simulink model "main"  (R2019b)
settings: Solver=VariableStepAuto  StartTime=0.0  StopTime=3  RelTol=1e-6  EnableMultiTasking=on
values from neighbouring files (symbols this model uses):
  gamma = 1.4    [main.m]
  M = kron(eye(N),C)    [MpcVectorize.m]    (also in MpcVectorizeLinearized.m; main.m = [0 1 0; 0 0 0])
  m = 1    [main.m]
  N = 20    [main.m]
  n = 3    [main.m]
  PI_Linear = 0.99    [main.m]
  q1 = [1e8 0; 0 0]    [main.m]
  q2 = 1e-8    (= 1e-08)    [main.m]
  Ts = 0.01    [main.m]
  x0 = [0.177; 2e4; 0]    [main.m]
  x0_plant = [0.177; 2e4]    [main.m]
undefined symbols (not defined in the file or in its folder): ENGINE, PI_Input
libraries: simulink x1, powerlib_meascontrol x1
settings Model: Creator=Robin  LastModifiedBy=geoja551
settings DataIOCC: ReturnWorkspaceOutputs=off
settings OptimizationCC: LifeSpan=inf
settings DebuggingCC: SFUnexpectedBacktrackingDiag=warning  SFNoUnconditionalDefaultTransitionDiag=warning  UnderSpecifiedDimensionMsg=warning  ArithmeticOperatorsInVariantConditions=warning
settings SFSimCC: SimUseLocalCustomCode=off  CustomCodeUndefinedFunction=UseInterfaceOnly
settings RTWCC: RTWUseLocalCustomCode=off
settings CodeAppCC: StateflowObjectComments=on
settings GRTTargetCC: TargetLangStandard=C89/C90 (ANSI)  GeneratePreprocessorConditionals=Disable all
settings ConfigComp: CovMetricSettings=dw  CovHtmlReporting=on  CovSaveCumulativeToWorkspaceVar=on  CovSaveSingleToWorkspaceVar=on  CovExternalEMLEnable=off

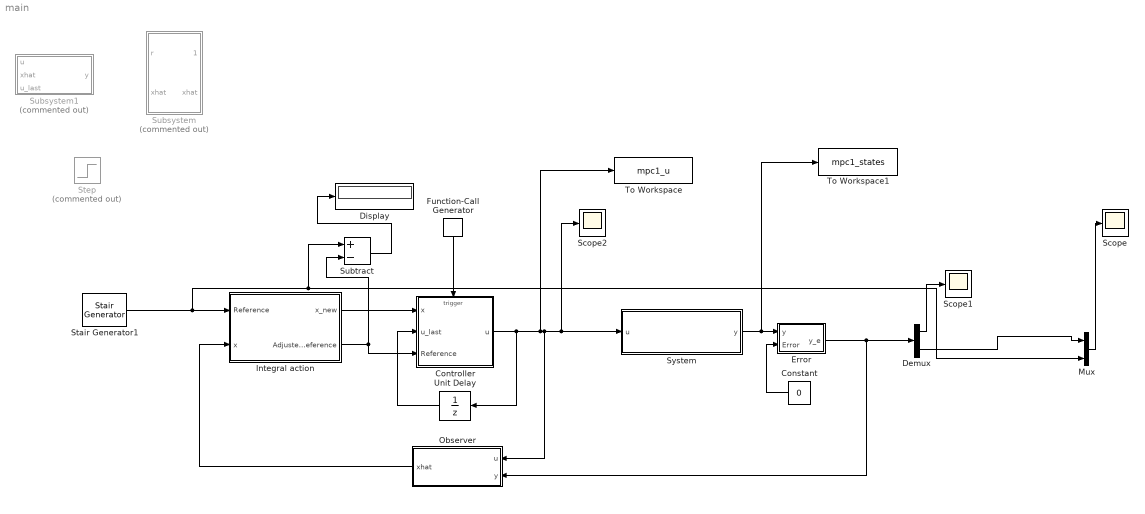
== system main ==
  Constant : Constant  Value=0
  Controller : Subsystem
  Demux : Demux  Outputs=2
  Display : Display
  Error : Subsystem
  Function-Call Generator : simulink/Ports & Subsystems/Function-Call Generator  sample_time=Ts  numberOfIterations=1
  Integral action : Subsystem
  Mux : Mux  Inputs=2
  Observer : Subsystem
  Scope : Scope
  Scope1 : Scope
  Scope2 : Scope
  Stair Generator1 : powerlib_meascontrol/Pulse & Signal Generators/Stair Generator  t=[0,1]  e=[ 2e4,8e4]  Ts=0
      settings: SourceProductName=Simscape Electrical
  Step : Step  Commented=on  Time=4  Before=2e4  After=6e4  SampleTime=0
  Subsystem : Subsystem  Commented=on
  Subsystem1 : Subsystem  Commented=on
  Subtract : Sum  Inputs=+-
  System : Subsystem
  To Workspace : ToWorkspace  VariableName=mpc1_u  SaveFormat=Structure With Time  SampleTime=-1
  To Workspace1 : ToWorkspace  VariableName=mpc1_states  SaveFormat=Structure With Time  SampleTime=-1
  Unit Delay : UnitDelay  InitialCondition=x0(1)  SampleTime=Ts  HasFrameUpgradeWarning=on
  wires:
  Function-Call Generator/1 -> Controller/Trigger
  Unit Delay/1 -> Controller/2(u_last)
  Controller/1(u) -> To Workspace/1, Scope2/1, System/1(u), Observer/1(u), Unit Delay/1
  System/1(y) -> To Workspace1/1, Error/1(y)
  Error/1(y_e) -> Demux/1, Observer/2(y)
  Constant/1 -> Error/2(Error)
  Integral action/2(Adjusted Reference) -> Subtract/2, Controller/3(Reference)
  Observer/1(xhat) -> Integral action/2(x)
  Integral action/1(x_new) -> Controller/1(x)
  Demux/2 -> Mux/1
  Demux/1 -> Scope1/1
  Mux/1 -> Scope/1
  Stair Generator1/1 -> Subtract/1, Mux/2, Integral action/1(Reference)
  Subtract/1 -> Display/1

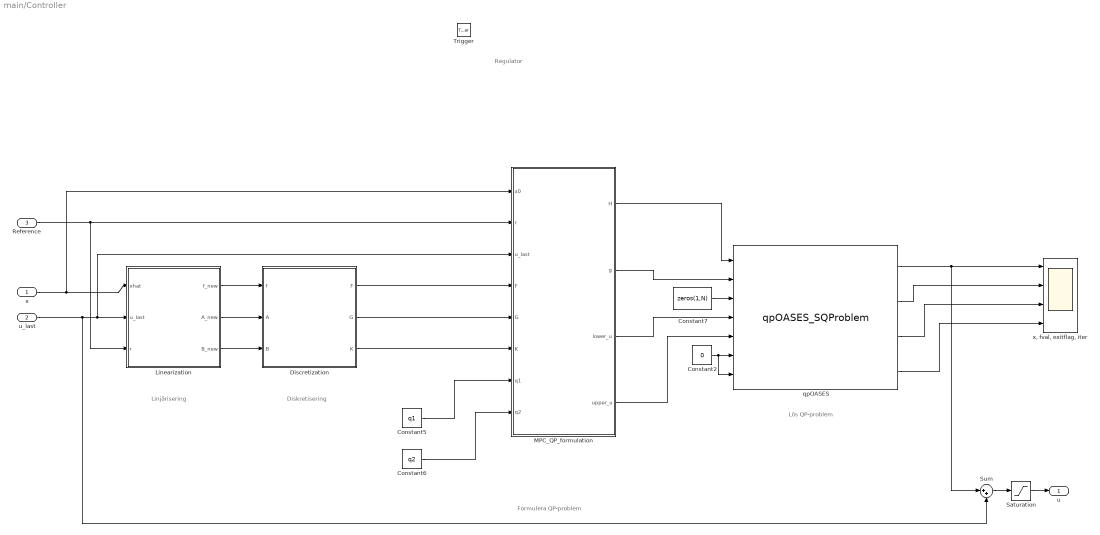
== system main/Controller ==
  note: Diskretisering
  note: Regulator
  note: Formulera QP-problem
  note: Lös QP-problem
  note: Linjärisering
  x : Inport
  u_last : Inport  Port=2  PortDimensions=1
  Reference : Inport  Port=3
  Trigger : TriggerPort  TriggerType=function-call  VariantControl=Variant  PortDimensions=1
  Constant2 : Constant  Value=0
  Constant5 : Constant  Value=q1
  Constant6 : Constant  Value=q2
  Constant7 : Constant  Value=zeros(1,N)
  Discretization : MATLAB Function  TreatAsAtomicUnit=on
  Linearization : MATLAB Function  TreatAsAtomicUnit=on
  MPC_QP_formulation : MATLAB Function  TreatAsAtomicUnit=on
  Saturation : Saturate  UpperLimit=1  LowerLimit=0
  Sum : Sum  Inputs=|++
  qpOASES : S-Function  FunctionName=qpOASES_SQProblem  SFunctionDeploymentMode=off  EnableBusSupport=off
  "x, fval, exitflag, iter" : Scope  NumInputPorts=4
  u : Outport
  wires:
  Linearization/2(A_new) -> Discretization/2(A)
  Linearization/3(B_new) -> Discretization/3(B)
  Discretization/1(F) -> MPC_QP_formulation/4(F)
  Discretization/2(G) -> MPC_QP_formulation/5(G)
  Constant6/1 -> MPC_QP_formulation/8(q2)
  Constant5/1 -> MPC_QP_formulation/7(q1)
  qpOASES/1 -> Sum/1, "x, fval, exitflag, iter"/1
  qpOASES/2 -> "x, fval, exitflag, iter"/2
  qpOASES/3 -> "x, fval, exitflag, iter"/3
  qpOASES/4 -> "x, fval, exitflag, iter"/4
  MPC_QP_formulation/2(g) -> qpOASES/2
  Constant7/1 -> qpOASES/3
  MPC_QP_formulation/3(lower_u) -> qpOASES/4
  MPC_QP_formulation/4(upper_u) -> qpOASES/5
  MPC_QP_formulation/1(H) -> qpOASES/1
  Constant2/1 -> qpOASES/7, qpOASES/6
  x/1 -> MPC_QP_formulation/1(x0), Linearization/1(xhat)
  u_last/1 -> Sum/2, Linearization/2(u_last), MPC_QP_formulation/3(u_last)
  Discretization/3(K) -> MPC_QP_formulation/6(K)
  Reference/1 -> Linearization/3(r), MPC_QP_formulation/2(r)
  Linearization/1(f_new) -> Discretization/1(f)
  Saturation/1 -> u/1
  Sum/1 -> Saturation/1

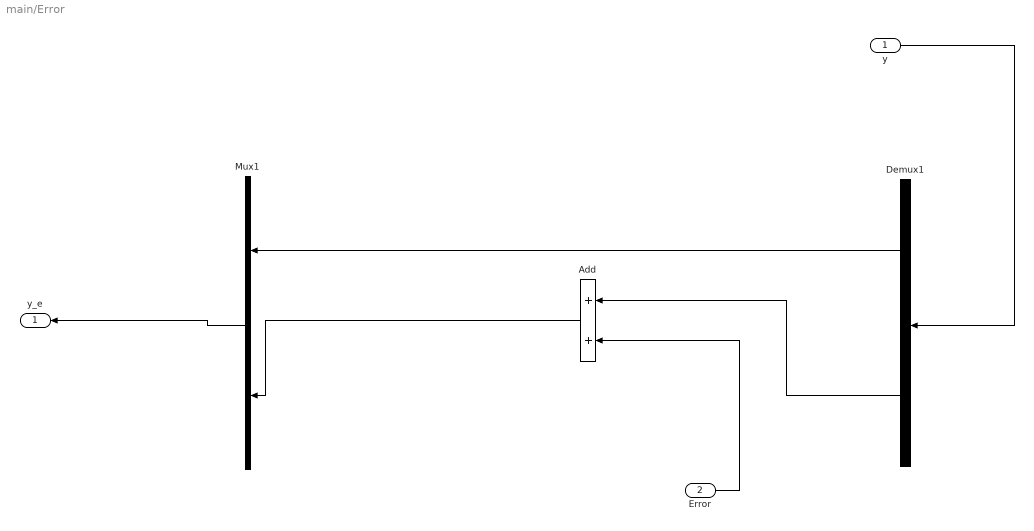
== system main/Error ==
  y : Inport
  Error : Inport  Port=2
  Add : Sum
  Demux1 : Demux  Outputs=2
  Mux1 : Mux  Inputs=2
  y_e : Outport
  wires:
  y/1 -> Demux1/1
  Mux1/1 -> y_e/1
  Demux1/2 -> Add/1
  Add/1 -> Mux1/2
  Demux1/1 -> Mux1/1
  Error/1 -> Add/2

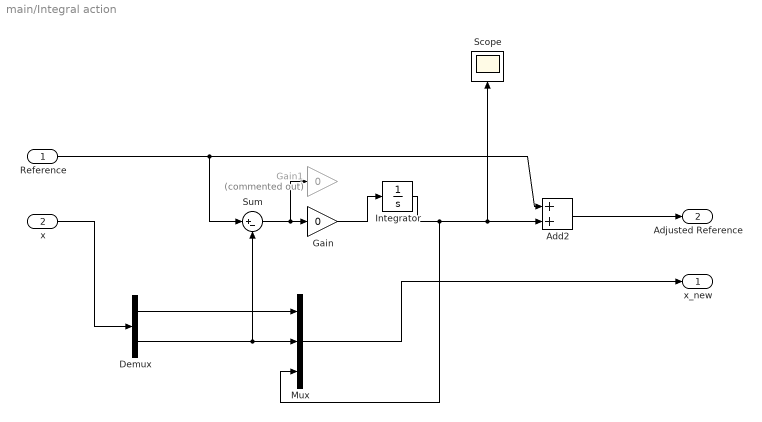
== system main/Integral action ==
  Reference : Inport
  x : Inport  Port=2
  Add2 : Sum
  Demux : Demux  Outputs=2
  Gain : Gain  Gain=0
  Gain1 : Gain  Commented=on  Gain=0
  Integrator : Integrator
  Mux : Mux  Inputs=3
  Scope : Scope
  Sum : Sum  Inputs=|+-
  x_new : Outport
  Adjusted Reference : Outport  Port=2
  wires:
  Add2/1 -> Adjusted Reference/1
  Reference/1 -> Sum/1, Add2/1
  x/1 -> Demux/1
  Demux/1 -> Mux/1
  Demux/2 -> Sum/2, Mux/2
  Sum/1 -> Gain1/1, Gain/1
  Mux/1 -> x_new/1
  Integrator/1 -> Mux/3, Add2/2, Scope/1
  Gain/1 -> Integrator/1

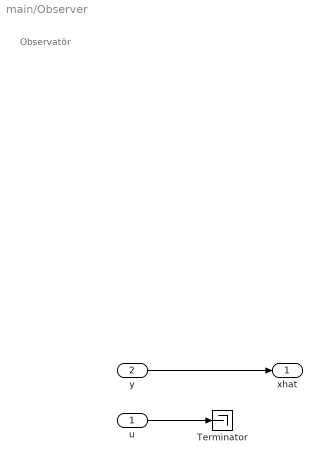
== system main/Observer ==
  note: Observatör
  u : Inport
  y : Inport  Port=2
  Terminator : Terminator
  xhat : Outport
  wires:
  u/1 -> Terminator/1
  y/1 -> xhat/1

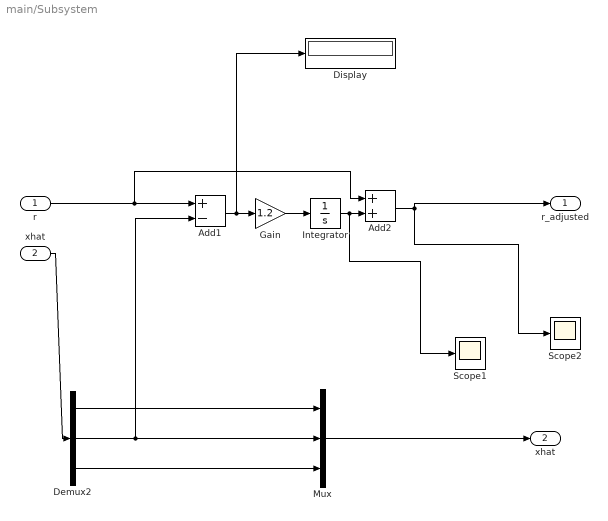
== system main/Subsystem ==
  r : Inport
  xhat : Inport  Port=2
  Add1 : Sum  Inputs=+-
  Add2 : Sum
  Demux2 : Demux  Outputs=3
  Display : Display
  Gain : Gain  Gain=1.2
  Integrator : Integrator
  Mux : Mux  Inputs=3
  Scope1 : Scope
  Scope2 : Scope
  r_adjusted : Outport
  "xhat " : Outport  Port=2
  wires:
  Add1/1 -> Display/1, Gain/1
  Gain/1 -> Integrator/1
  Add2/1 -> Scope2/1, r_adjusted/1
  Integrator/1 -> Scope1/1, Add2/2
  r/1 -> Add2/1, Add1/1
  xhat/1 -> Demux2/1
  Mux/1 -> "xhat "/1
  Demux2/1 -> Mux/1
  Demux2/2 -> Mux/2, Add1/2
  Demux2/3 -> Mux/3

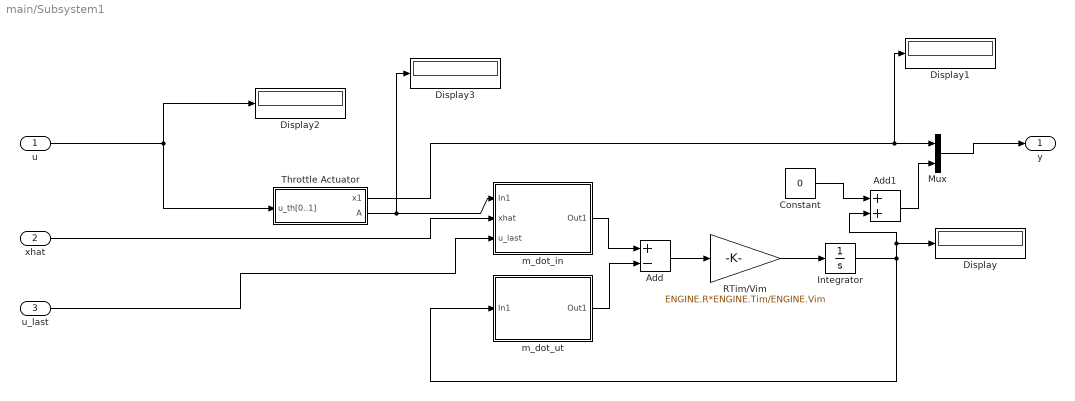
== system main/Subsystem1 ==
  u : Inport
  "xhat " : Inport  Port=2
  u_last : Inport  Port=3
  Add : Sum  Inputs=+-
  Add1 : Sum
  Constant : Constant  Value=0
  Display{,1..3} (4 alike) : Display
  Integrator : Integrator  InitialCondition=25000
  Mux : Mux  Inputs=2
  RTim/Vim : Gain  Gain=ENGINE.R*ENGINE.Tim/ENGINE.Vim
  Throttle Actuator : Subsystem
  m_dot_in : Subsystem
  m_dot_ut : Subsystem
  y : Outport  PortDimensions=2  VectorParamsAs1DForOutWhenUnconnected=off
  wires:
  u/1 -> Display2/1, Throttle Actuator/1(u_th[0..1])
  Throttle Actuator/1("x1 ") -> Display1/1, Mux/1
  Add/1 -> RTim/Vim/1
  RTim/Vim/1 -> Integrator/1
  Integrator/1 -> Add1/2, Display/1, m_dot_ut/1(In1)
  Throttle Actuator/2("A ") -> Display3/1, m_dot_in/1(In1)
  m_dot_in/1(Out1) -> Add/1
  m_dot_ut/1(Out1) -> Add/2
  Mux/1 -> y/1
  Add1/1 -> Mux/2
  Constant/1 -> Add1/1
  "xhat "/1 -> m_dot_in/2(xhat)
  u_last/1 -> m_dot_in/3(u_last)

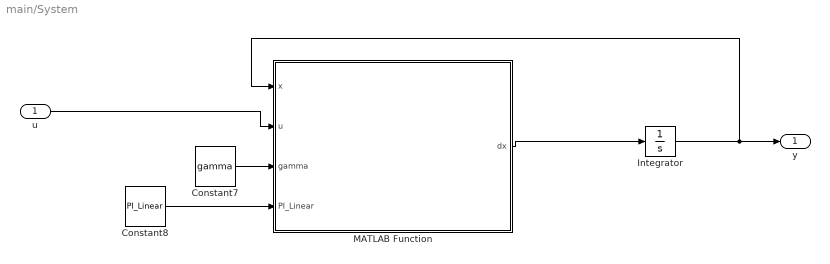
== system main/System ==
  u : Inport
  Constant7 : Constant  Value=gamma
  Constant8 : Constant  Value=PI_Linear
  Integrator : Integrator  InitialCondition=x0_plant
  MATLAB Function : MATLAB Function  TreatAsAtomicUnit=on
  y : Outport
  wires:
  u/1 -> MATLAB Function/2(u)
  MATLAB Function/1(dx) -> Integrator/1
  Integrator/1 -> MATLAB Function/1(x), y/1
  Constant7/1 -> MATLAB Function/3(gamma)
  Constant8/1 -> MATLAB Function/4(PI_Linear)

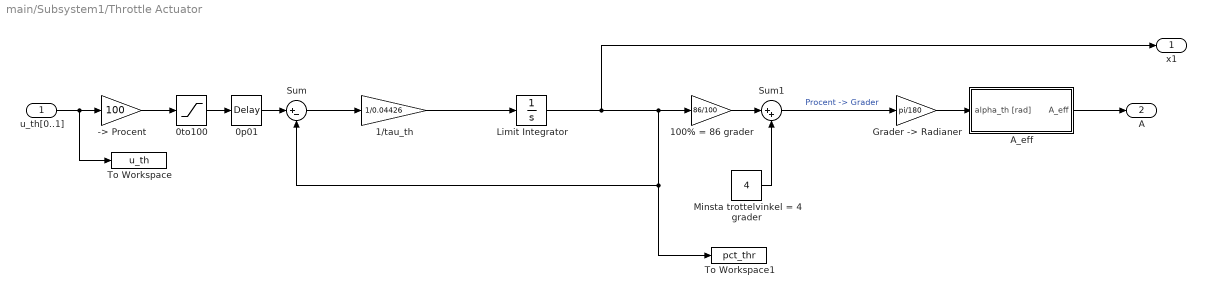
== system main/Subsystem1/Throttle Actuator ==
  u_th[0..1] : Inport
  -> Procent : Gain  Gain=100
  0p01 : TransportDelay  DelayTime=0.02
  0to100 : Saturate  UpperLimit=100  LowerLimit=0
  1/tau_th : Gain  Gain=1/0.04426
  100% = 86 grader : Gain  Gain=86/100
  A_eff : Subsystem
  "Grader -> Radianer" : Gain  Gain=pi/180
  Limit Integrator : Integrator  LimitOutput=on  UpperSaturationLimit=100  LowerSaturationLimit=0
  Minsta trottelvinkel = 4 grader : Constant  Value=4
  Sum : Sum  Inputs=|+-
  Sum1 : Sum  Inputs=|++
  To Workspace : ToWorkspace  VariableName=u_th  SampleTime=-1
  To Workspace1 : ToWorkspace  VariableName=pct_thr  SampleTime=-1
  "x1 " : Outport  VectorParamsAs1DForOutWhenUnconnected=off
  "A " : Outport  Port=2  VectorParamsAs1DForOutWhenUnconnected=off
  wires:
  Sum/1 -> 1/tau_th/1
  Limit Integrator/1 -> "x1 "/1, 100% = 86 grader/1, To Workspace1/1, Sum/2
  1/tau_th/1 -> Limit Integrator/1
  0to100/1 -> 0p01/1
  0p01/1 -> Sum/1
  u_th[0..1]/1 -> To Workspace/1, -> Procent/1
  Minsta trottelvinkel = 4 grader/1 -> Sum1/2
  100% = 86 grader/1 -> Sum1/1
  Sum1/1 -> "Grader -> Radianer"/1  "Procent -> Grader"
  "Grader -> Radianer"/1 -> A_eff/1(alpha_th [rad])
  -> Procent/1 -> 0to100/1
  A_eff/1(A_eff) -> "A "/1

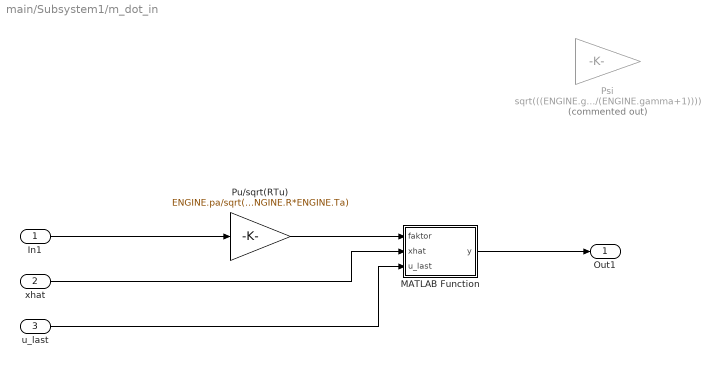
== system main/Subsystem1/m_dot_in ==
  In1 : Inport
  xhat : Inport  Port=2
  u_last : Inport  Port=3
  MATLAB Function : MATLAB Function  TreatAsAtomicUnit=on
  Psi : Gain  Commented=on  Gain=sqrt(((ENGINE.gamma+1)/(2*ENGINE.gamma))*(1-PI_Input)*(PI_Input+((ENGINE.gamma-1)/(ENGINE.gamma+1))))
  Pu/sqrt(RTu) : Gain  Gain=ENGINE.pa/sqrt(ENGINE.R*ENGINE.Ta)
  Out1 : Outport  VectorParamsAs1DForOutWhenUnconnected=off
  wires:
  In1/1 -> Pu/sqrt(RTu)/1
  Pu/sqrt(RTu)/1 -> MATLAB Function/1(faktor)
  MATLAB Function/1(y) -> Out1/1
  xhat/1 -> MATLAB Function/2(xhat)
  u_last/1 -> MATLAB Function/3(u_last)

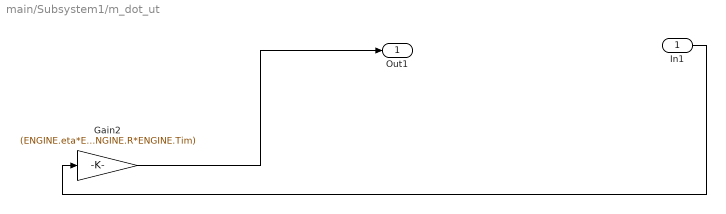
== system main/Subsystem1/m_dot_ut ==
  In1 : Inport
  Gain2 : Gain  Gain=(ENGINE.eta*ENGINE.Vd*ENGINE.N)/(ENGINE.nr*ENGINE.R*ENGINE.Tim)
  Out1 : Outport  VectorParamsAs1DForOutWhenUnconnected=off
  wires:
  Gain2/1 -> Out1/1
  In1/1 -> Gain2/1

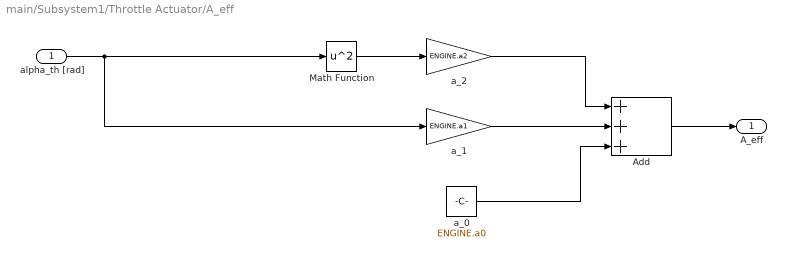
== system main/Subsystem1/Throttle Actuator/A_eff ==
  alpha_th [rad] : Inport
  Add : Sum  Inputs=+++
  Math Function : Math  Operator=square  SaturateOnIntegerOverflow=on
  a_0 : Constant  Value=ENGINE.a0
  a_1 : Gain  Gain=ENGINE.a1
  a_2 : Gain  Gain=ENGINE.a2
  A_eff : Outport  VectorParamsAs1DForOutWhenUnconnected=off
  wires:
  Math Function/1 -> a_2/1
  a_2/1 -> Add/1
  a_1/1 -> Add/2
  a_0/1 -> Add/3
  Add/1 -> A_eff/1
  alpha_th [rad]/1 -> Math Function/1, a_1/1

== matlab function main/Controller/Linearization ==
  data: f_new output; xhat input; A_new output; u_last input; B_new output; gamma parameter; r input; x0 parameter
function [f_new,A_new,B_new] = fcn(xhat,u_last,gamma,r,x0)
PI_Input = PI_function(xhat, u_last);
PI_Critical = 1/(gamma+1);

A_shell = zeros(3,3);
B_shell = zeros(3,1);
f_shell = zeros(3,1);
    if PI_Input < PI_Critical
        A = mpcControllerA_1(xhat,u_last);
        B = mpcControllerB_1(xhat,u_last);
        f = mpcControllerf_1(xhat,u_last);
    elseif PI_Input <= 0.99
        A = mpcControllerA_2(xhat,u_last);
        B = mpcControllerB_2(xhat,u_last);
        f = mpcControllerf_2(xhat,u_last);
    else
        A = mpcControllerA_3(xhat,u_last);
        B = mpcControllerB_3(xhat,u_last);
        f = mpcControllerf_3(xhat,u_last);
    end
A_shell(1:2,1:2)= A(1:2,1:2);
A_shell(3,3) = -1;
B_shell(1:2) = B(1:2);
B_shell(3) = 0;
f_shell(1:2) = f(1:2);
f_shell(3) = (r - xhat(3));
A_new = A_shell;
B_new = B_shell;
f_new = f_shell;
end

== matlab function main/Controller/Discretization ==
  data: f input; A input; F output; B input; G output; Ts parameter; K output
% x_k+1 = x_k + Ts*(Ax_k+Bu_k) = [I+Ts*A]*x_k + Ts*B*u_k
% F = [I+Ts*A]
% G = Ts*B
function [F,G,K] = Discretize(f,A,B,Ts)
    F = eye(size(A))+Ts*A;
    G = Ts*B;
    K = Ts*f;
end

== matlab function main/Controller/MPC_QP_formulation ==
  data: x0 input; r input; u_last input; F input; H output; G input; K input; g output; q1 input; q2 input; lower_u output; upper_u output; n parameter; m parameter; N parameter; M parameter
function [H,g,lower_u,upper_u] = MPC_vectorize(x0,r,u_last,F,G,K,q1,q2,n, m, N, M)
    H = zeros(m^2*N^2,1);
    
    constraint_upper = 1; % Set upper constraint for u
    constraint_lower = 0; % Set upper constraint for u
    lower_u = (constraint_lower-u_last)*ones(N,1);
    upper_u = (constraint_upper-u_last)*ones(N,1);
    
    x0 = repmat(x0,[N,1]);
    U0 = repmat(u_last,[N,1]);
    
    % Generate the G matrix on p. 158 Industriell Reglerteknik
    % Generate the M,Q1, and Q2 matrix on p. 159 Industriell Reglerteknik
    [G,D,M] = MpcVectorizeLinearized(F,G,M,K,N,m,n);
    Q1 = CreateBlockDiagonal(q1,N);
    Q2 = CreateBlockDiagonal(q2,N);
    % Omega = eye(N*m) - [zeros(m,N*m); eye((N-1)*m) zeros((N-1)*m,m)];
    % delta = [u_last; zeros((N-1)*m,1)];

    % Generate reference signal, this assumes the r-value for the
    % prediction horizon.
    ref_sig = [r*ones(N,1); zeros(N,1)];
    
    % Generate H matrix as (10.15a) p. 159 Industriell Reglerteknik with
    % cost-function as (10.22). So with reference following.
    [H_temp, g_temp] = MpcQPformulationLinearized(G,M,D);
    H_temp = H_temp(Q1,Q2);
    g_temp = g_temp(x0,Q1,Q2,U0,ref_sig);
    
    % qpOASES needs flat vectors as input. (not verified with two inputs.)
    H(:) = H_temp(:);
    g = g_temp(:);
end

== matlab function main/Subsystem1/m_dot_in/MATLAB Function ==
  data: faktor input; y output; xhat input; u_last input; gamma parameter
function y = fcn(faktor,xhat,u_last,gamma)
PIL=0.99;
PI_Input = PI(xhat, u_last);
if (PI_Input >= 1/(gamma+1) && PI_Input <= 0.99 )
    y = faktor*mpcControllerPSI_standard(xhat,u_last);
    PI_Used = ('Standard PI');
elseif (PI_Input > 0.99)
    y = faktor*( sqrt(((2*gamma)/(gamma-1))...
    *((PIL^(2/gamma))-(PIL^((gamma+1)...
    /(gamma))))));
    PI_Used = ('Linear PI');
else
    y = faktor*( sqrt(((gamma+1)/(2*gamma))...
    *(1-(1/(gamma+1)))*((1/(gamma+1))+((gamma-1)...
    /(gamma+1)))));
    PI_Used = ('Otherwise PI');
end 
end

== matlab function main/System/MATLAB Function ==
  data: x input; u input; dx output; gamma input; PI_Linear input
function dx = fcn(x,u,gamma,PI_Linear)
PI_Input = PI_function(x,u);
PI_Critical = 1/(gamma+1);

    if PI_Input < PI_Critical
        dx = mpcControllerf_plant_1(x,u);
    elseif PI_Input <= PI_Linear
        dx = mpcControllerf_plant_2(x,u);
    else
        dx = mpcControllerf_plant_3(x,u);
    end
end
